simulink model "EGRVlv_VDPosGov"  (R2016b)
settings: configuration reference "CodeGenConfigSet" (kept outside this file)
values from neighbouring files (symbols this model uses):
  EGRVlv_ctClnUpFin_C = Calibration.Parameter    [init_EGRVlv_VDPosGov.m]
  EGRVlv_DKdNgv_C = Calibration.Parameter    [init_EGRVlv_VDPosGov.m]
  EGRVlv_DKdPsv_C = Calibration.Parameter    [init_EGRVlv_VDPosGov.m]
  EGRVlv_drActNgv_C = Calibration.Parameter    [init_EGRVlv_VDPosGov.m]
  EGRVlv_facCrntEffFlt_C = Calibration.Parameter    [init_EGRVlv_VDPosGov.m]
  EGRVlv_iEff_CUR = Calibration.Parameter    [init_EGRVlv_VDPosGov.m]
  EGRVlv_iEff_CURX = Calibration.Parameter    [init_EGRVlv_VDPosGov.m]
  EGRVlv_iEffOvrLd_C = Calibration.Parameter    [init_EGRVlv_VDPosGov.m]
  EGRVlv_IKiLMSSlp_C = Calibration.Parameter    [init_EGRVlv_VDPosGov.m]
  EGRVlv_IKiNgv_C = Calibration.Parameter    [init_EGRVlv_VDPosGov.m]
  EGRVlv_IKiPsv_C = Calibration.Parameter    [init_EGRVlv_VDPosGov.m]
  EGRVlv_KdParDT1_C = Calibration.Parameter    [init_EGRVlv_VDPosGov.m]
  EGRVlv_PKpNgv_C = Calibration.Parameter    [init_EGRVlv_VDPosGov.m]
  EGRVlv_PKpPsv_C = Calibration.Parameter    [init_EGRVlv_VDPosGov.m]
  EGRVlv_rActNgv_C = Calibration.Parameter    [init_EGRVlv_VDPosGov.m]
  EGRVlv_rDesClnUpCls_C = Calibration.Parameter    [init_EGRVlv_VDPosGov.m]
  EGRVlv_rDesClnUpOpen_C = Calibration.Parameter    [init_EGRVlv_VDPosGov.m]
  EGRVlv_rDesEGR_CUR = Calibration.Parameter    [init_EGRVlv_VDPosGov.m]
  EGRVlv_rDesEGR_CURX = Calibration.Parameter    [init_EGRVlv_VDPosGov.m]
  EGRVlv_rDesLMSMin_C = Calibration.Parameter    [init_EGRVlv_VDPosGov.m]
  EGRVlv_rDesOffHold_C = Calibration.Parameter    [init_EGRVlv_VDPosGov.m]
  EGRVlv_rEGRDflVal_C = Calibration.Parameter    [init_EGRVlv_VDPosGov.m]
  EGRVlv_rEGRSwtOff_C = Calibration.Parameter    [init_EGRVlv_VDPosGov.m]
  EGRVlv_rGovDvtThres_C = Calibration.Parameter    [init_EGRVlv_VDPosGov.m]
  EGRVlv_rGovMax_C = Calibration.Parameter    [init_EGRVlv_VDPosGov.m]
  EGRVlv_rGovMax_CUR = Calibration.Parameter    [init_EGRVlv_VDPosGov.m]
  EGRVlv_rGovMax_CURX = Calibration.Parameter    [init_EGRVlv_VDPosGov.m]
  EGRVlv_rGovMin_C = Calibration.Parameter    [init_EGRVlv_VDPosGov.m]
  EGRVlv_rGovMin_CUR = Calibration.Parameter    [init_EGRVlv_VDPosGov.m]
  EGRVlv_rGovMin_CURX = Calibration.Parameter    [init_EGRVlv_VDPosGov.m]
  EGRVlv_rIniStp_C = Calibration.Parameter    [init_EGRVlv_VDPosGov.m]
  EGRVlv_rOutDMax_C = Calibration.Parameter    [init_EGRVlv_VDPosGov.m]
  EGRVlv_rOutIMax_C = Calibration.Parameter    [init_EGRVlv_VDPosGov.m]
  EGRVlv_rPIDWinNgv_C = Calibration.Parameter    [init_EGRVlv_VDPosGov.m]
  EGRVlv_rPIDWinPsv_C = Calibration.Parameter    [init_EGRVlv_VDPosGov.m]
  EGRVlv_rSwtOffRmp_C = Calibration.Parameter    [init_EGRVlv_VDPosGov.m]
  EGRVlv_SlwClsDKd_C = Calibration.Parameter    [init_EGRVlv_VDPosGov.m]
  EGRVlv_SlwClsIKi_C = Calibration.Parameter    [init_EGRVlv_VDPosGov.m]
  EGRVlv_SlwClsPKp_C = Calibration.Parameter    [init_EGRVlv_VDPosGov.m]
  EGRVlv_SmlSigNgvDKd_C = Calibration.Parameter    [init_EGRVlv_VDPosGov.m]
  EGRVlv_SmlSigNgvIKi_C = Calibration.Parameter    [init_EGRVlv_VDPosGov.m]
  EGRVlv_SmlSigNgvPKp_C = Calibration.Parameter    [init_EGRVlv_VDPosGov.m]
  EGRVlv_SmlSigPsvDKd_C = Calibration.Parameter    [init_EGRVlv_VDPosGov.m]
  EGRVlv_SmlSigPsvIKi_C = Calibration.Parameter    [init_EGRVlv_VDPosGov.m]
  EGRVlv_SmlSigPsvPKp_C = Calibration.Parameter    [init_EGRVlv_VDPosGov.m]
  EGRVLV_STCLNUP_CLOSE = fi(3,State_uint8)    [init_EGRVlv_VDPosGov.m]
  EGRVLV_STCLNUP_FINISH = fi(4,State_uint8)    [init_EGRVlv_VDPosGov.m]
  EGRVLV_STCLNUP_INIT = fi(1,State_uint8)    [init_EGRVlv_VDPosGov.m]
  EGRVLV_STCLNUP_OPEN = fi(2,State_uint8)    [init_EGRVlv_VDPosGov.m]
  EGRVlv_stClnUpInh_C = Calibration.Parameter    [init_EGRVlv_VDPosGov.m]
  EGRVlv_swtDesValNrmInv_C = Calibration.Parameter    [init_EGRVlv_VDPosGov.m]
  EGRVlv_swtEGRTyp_C = Calibration.Parameter    [init_EGRVlv_VDPosGov.m]
  EGRVlv_swtGovByp_C = Calibration.Parameter    [init_EGRVlv_VDPosGov.m]
  EGRVlv_swtSelDT1In_C = Calibration.Parameter    [init_EGRVlv_VDPosGov.m]
  EGRVlv_tiClnUp_C = Calibration.Parameter    [init_EGRVlv_VDPosGov.m]
  EGRVlv_tiGovDT1_C = Calibration.Parameter    [init_EGRVlv_VDPosGov.m]
  EGRVlv_tiLimDlyOvrLd_C = Calibration.Parameter    [init_EGRVlv_VDPosGov.m]
  EGRVlv_tiOutIMax_C = Calibration.Parameter    [init_EGRVlv_VDPosGov.m]
  EGRVlv_tiParDT1_C = Calibration.Parameter    [init_EGRVlv_VDPosGov.m]
  MINUS_1_PRC = fi(-1,Prc_100_rate)    [init_EGRVlv_VDPosGov.m]
  RLS = fi(0,State_uint8)    [init_EGRVlv_VDPosGov.m]
  VALEO = fi(0,State_uint8)    [init_EGRVlv_VDPosGov.m]
  ZERO_PRC = fi(0,Prc_100_rate)    [init_EGRVlv_VDPosGov.m]
undefined symbols (not defined in the file or in its folder): CEngDsT_tTransf_CURX, EGRVlv_VDPosGov_DT, SubSysExeState_conv
libraries: CXLib x32, simulink x12
(part 2 of 2)

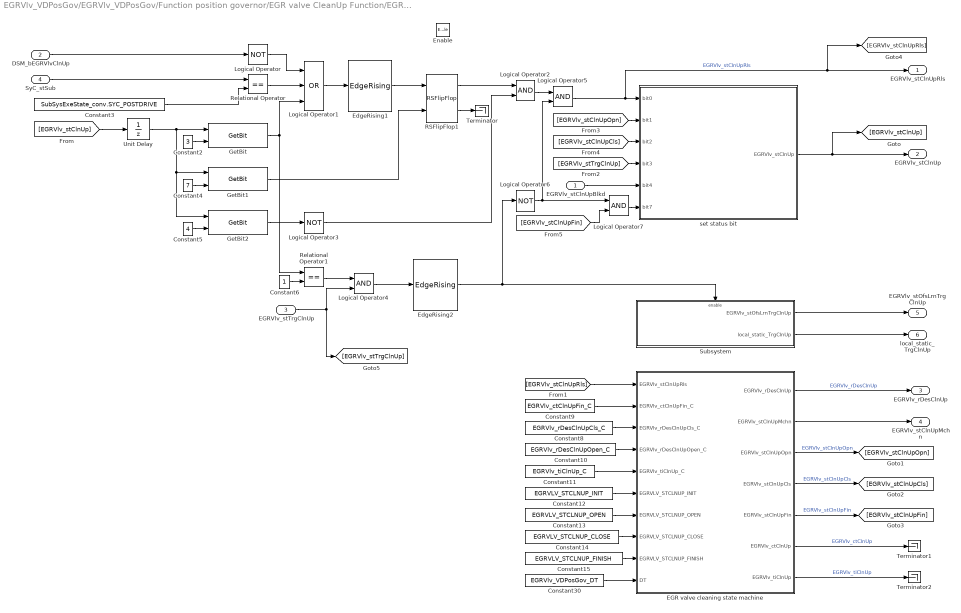
== system EGRVlv_VDPosGov/EGRVlv_VDPosGov/Function position governor/EGR valve CleanUp Function/EGR valve CleanUp release conditions ==
  EGRVlv_stClnUpBlkd : Inport
  DSM_bEGRVlvClnUp : Inport  Tag=%  Port=2
  EGRVlv_stTrgClnUp : Inport  Port=3
  SyC_stSub : Inport  Tag=%  Port=4
  Enable : EnablePort
  Constant10 : Constant  Value=EGRVlv_rDesClnUpOpen_C
  Constant11 : Constant  Value=EGRVlv_tiClnUp_C
  Constant12 : Constant  Value=EGRVLV_STCLNUP_INIT
  Constant13 : Constant  Value=EGRVLV_STCLNUP_OPEN
  Constant14 : Constant  Value=EGRVLV_STCLNUP_CLOSE
  Constant15 : Constant  Value=EGRVLV_STCLNUP_FINISH
  Constant2 : Constant  Value=3  OutDataTypeStr=uint8
  Constant3 : Constant  Value=SubSysExeState_conv.SYC_POSTDRIVE  OutDataTypeStr=Enum:SubSysExeState_conv
  Constant30 : Constant  Value=EGRVlv_VDPosGov_DT
  Constant4 : Constant  Value=7  OutDataTypeStr=uint8
  Constant5 : Constant  Value=4  OutDataTypeStr=uint8
  Constant6 : Constant  OutDataTypeStr=uint8
  Constant8 : Constant  Value=EGRVlv_rDesClnUpCls_C
  Constant9 : Constant  Value=EGRVlv_ctClnUpFin_C
  EGR valve cleaning state machine : Stateflow chart  TreatAsAtomicUnit=on
  EdgeRising1 : CXLib/EdgeRising
  EdgeRising2 : CXLib/EdgeRising
  GetBit : CXLib/GetBit  dataTypeString=uint8  dataLength=0
      settings: AttributesFormatString=Get bit from %<dataTypeString>
  GetBit1 : CXLib/GetBit  dataTypeString=uint8  dataLength=0
      settings: AttributesFormatString=Get bit from %<dataTypeString>
  GetBit2 : CXLib/GetBit  dataTypeString=uint8  dataLength=0
      settings: AttributesFormatString=Get bit from %<dataTypeString>
  Logical Operator : Logic  Operator=NOT  AllPortsSameDT=off  OutDataTypeStr=boolean
  Logical Operator1 : Logic  Operator=OR  Inputs=3  AllPortsSameDT=off  OutDataTypeStr=boolean
  Logical Operator{2,4..5,7} (4 alike) : Logic  AllPortsSameDT=off  OutDataTypeStr=boolean
  Logical Operator3 : Logic  Operator=NOT  AllPortsSameDT=off  OutDataTypeStr=boolean
  Logical Operator6 : Logic  Operator=NOT  AllPortsSameDT=off  OutDataTypeStr=boolean
  RSFlipFlop1 : CXLib/RSFlipFlop
  Relational Operator : RelationalOperator  Operator===  OutDataTypeStr=boolean  RndMeth=Simplest
  Relational Operator1 : RelationalOperator  Operator===  OutDataTypeStr=boolean  RndMeth=Simplest
  Subsystem : Subsystem
  Terminator : Terminator
  Terminator1 : Terminator
  Terminator2 : Terminator
  Unit Delay : UnitDelay  SampleTime=-1
      settings: AttributesFormatString=InitialValue=%<InitialCondition>
  set status bit : Subsystem
  EGRVlv_stClnUpRls : Outport  Tag=%
  EGRVlv_stClnUp : Outport  Tag=%  Port=2
  EGRVlv_rDesClnUp : Outport  Tag=%  Port=3
  EGRVlv_stClnUpMchn : Outport  Tag=%  Port=4
  EGRVlv_stOfsLrnTrgClnUp : Outport  Tag=%  Port=5
  local_static_TrgClnUp : Outport  Tag=%  Port=6
  wires:
  DSM_bEGRVlvClnUp/1 -> Logical Operator/1
  Logical Operator/1 -> Logical Operator1/1
  Logical Operator1/1 -> EdgeRising1/1
  EdgeRising1/1 -> RSFlipFlop1/1
  RSFlipFlop1/1 -> Logical Operator2/1
  Constant2/1 -> GetBit/2
  Constant3/1 -> Relational Operator/2
  SyC_stSub/1 -> Relational Operator/1
  GetBit/1 -> Logical Operator1/3, Relational Operator1/1
  Constant4/1 -> GetBit1/2
  GetBit1/1 -> RSFlipFlop1/2
  Constant5/1 -> GetBit2/2
  [EGRVlv_stClnUp] -> Unit Delay/1
  GetBit2/1 -> Logical Operator3/1
  Logical Operator3/1 -> Logical Operator2/2
  Relational Operator1/1 -> Logical Operator4/1
  Logical Operator4/1 -> EdgeRising2/1
  EdgeRising2/1 -> Subsystem/Enable, Logical Operator6/1
  EGRVlv_stTrgClnUp/1 -> [EGRVlv_stTrgClnUp], Logical Operator4/2
  Logical Operator2/1 -> Logical Operator5/1
  Constant6/1 -> Relational Operator1/2
  Logical Operator6/1 -> Logical Operator5/2, Logical Operator7/1
  Logical Operator5/1 -> [EGRVlv_stClnUpRls], EGRVlv_stClnUpRls/1, set status bit/1(bit0)  "EGRVlv_stClnUpRls"
  Constant9/1 -> EGR valve cleaning state machine/2(EGRVlv_ctClnUpFin_C)
  Constant8/1 -> EGR valve cleaning state machine/3(EGRVlv_rDesClnUpCls_C)
  Constant10/1 -> EGR valve cleaning state machine/4(EGRVlv_rDesClnUpOpen_C)
  Constant11/1 -> EGR valve cleaning state machine/5(EGRVlv_tiClnUp_C)
  Constant30/1 -> EGR valve cleaning state machine/10(DT)
  set status bit/1(EGRVlv_stClnUp) -> [EGRVlv_stClnUp], EGRVlv_stClnUp/1
  Logical Operator7/1 -> set status bit/6(bit7)
  [EGRVlv_stClnUpFin] -> Logical Operator7/2
  Constant12/1 -> EGR valve cleaning state machine/6(EGRVLV_STCLNUP_INIT)
  Constant13/1 -> EGR valve cleaning state machine/7(EGRVLV_STCLNUP_OPEN)
  Constant15/1 -> EGR valve cleaning state machine/9(EGRVLV_STCLNUP_FINISH)
  Constant14/1 -> EGR valve cleaning state machine/8(EGRVLV_STCLNUP_CLOSE)
  Relational Operator/1 -> Logical Operator1/2
  Unit Delay/1 -> GetBit/1, GetBit2/1, GetBit1/1
  [EGRVlv_stClnUpRls] -> EGR valve cleaning state machine/1(EGRVlv_stClnUpRls)
  [EGRVlv_stClnUpOpn] -> set status bit/2(bit1)
  [EGRVlv_stClnUpCls] -> set status bit/3(bit2)
  [EGRVlv_stTrgClnUp] -> set status bit/4(bit3)
  EGRVlv_stClnUpBlkd/1 -> set status bit/5(bit4)
  EGR valve cleaning state machine/1(EGRVlv_rDesClnUp) -> EGRVlv_rDesClnUp/1  "EGRVlv_rDesClnUp"
  EGR valve cleaning state machine/2(EGRVlv_stClnUpMchn) -> EGRVlv_stClnUpMchn/1
  EGR valve cleaning state machine/3(EGRVlv_stClnUpOpn) -> [EGRVlv_stClnUpOpn]  "EGRVlv_stClnUpOpn"
  EGR valve cleaning state machine/4(EGRVlv_stClnUpCls) -> [EGRVlv_stClnUpCls]  "EGRVlv_stClnUpCls"
  EGR valve cleaning state machine/5(EGRVlv_stClnUpFin) -> [EGRVlv_stClnUpFin]  "EGRVlv_stClnUpFin"
  EGR valve cleaning state machine/6(EGRVlv_ctClnUp) -> Terminator1/1  "EGRVlv_ctClnUp"
  EGR valve cleaning state machine/7(EGRVlv_tiClnUp) -> Terminator2/1  "EGRVlv_tiClnUp"
  RSFlipFlop1/2 -> Terminator/1
  Subsystem/1(EGRVlv_stOfsLrnTrgClnUp) -> EGRVlv_stOfsLrnTrgClnUp/1
  Subsystem/2(local_static_TrgClnUp) -> local_static_TrgClnUp/1

== system EGRVlv_VDPosGov/EGRVlv_VDPosGov/Function position governor/EGR valve CleanUp Function/Subsystem1 ==
  Enable : EnablePort
  Constant1 : Constant  Value=0  OutDataTypeStr=boolean
  Constant7 : Constant  OutDataTypeStr=boolean
  EGRVlv_stOfsLrnTrgClnUp : Outport  Tag=%
  local_static_TrgClnUp : Outport  Tag=%  Port=2
  wires:
  Constant1/1 -> local_static_TrgClnUp/1
  Constant7/1 -> EGRVlv_stOfsLrnTrgClnUp/1

== system EGRVlv_VDPosGov/EGRVlv_VDPosGov/Function position governor/I_comp/Calc ==
  note: %系数Q=Ki*T0/100
  note: [Dvt/s]
  note: [Dvt/ms]
  Dvt : Inport
  T0 : Inport  Port=2
  Ki : Inport  Port=3
  KiPos : Inport  Port=4
  KiNeg : Inport  Port=5
  WinPos : Inport  Port=6
  WinNeg : Inport  Port=7
  function : TriggerPort  TriggerType=function-call  VariantControl=Variant
  Constant1 : Constant  Value=100  OutDataTypeStr=uint32
  Data Store Read : DataStoreRead  DataStoreName=outputlast1
  Data Store Write : DataStoreWrite  DataStoreName=outputlast1
  Data Type Conversion11 : DataTypeConversion  SaturateOnIntegerOverflow=on
  Divide2 : Product  Inputs=*/  OutDataTypeStr=fixdt(1,32,2^-16,0)  RndMeth=Round  SaturateOnIntegerOverflow=on
  Product1 : Product  OutDataTypeStr=fixdt(1,32,2^-16,0)  RndMeth=Round  SaturateOnIntegerOverflow=on
  Product3 : Product  OutDataTypeStr=fixdt(1,32,2^-16,0)  RndMeth=Round  SaturateOnIntegerOverflow=on
  Relational Operator : RelationalOperator  Operator=>  OutDataTypeStr=boolean  RndMeth=Nearest  InputSameDT=on
  Relational Operator1 : RelationalOperator  Operator=<  OutDataTypeStr=boolean  RndMeth=Nearest  InputSameDT=on
  Sum : Sum  OutDataTypeStr=fixdt(1,32,2^-16,0)  RndMeth=Round  SaturateOnIntegerOverflow=on  InputSameDT=on
  Switch : Switch  Criteria=u2 ~= 0  SaturateOnIntegerOverflow=on  InputSameDT=on
  Switch1 : Switch  Criteria=u2 ~= 0  SaturateOnIntegerOverflow=on  InputSameDT=on
  Out : Outport
  wires:
  Product3/1 -> Sum/2
  Divide2/1 -> Product3/2
  Constant1/1 -> Divide2/2
  Product1/1 -> Divide2/1
  Data Type Conversion11/1 -> Out/1
  Sum/1 -> Data Type Conversion11/1, Data Store Write/1
  Dvt/1 -> Relational Operator1/1, Relational Operator/1, Product3/1
  Switch1/1 -> Product1/1
  T0/1 -> Product1/2
  WinNeg/1 -> Relational Operator1/2
  Ki/1 -> Switch/3
  Data Store Read/1 -> Sum/1
  Switch/1 -> Switch1/3
  WinPos/1 -> Relational Operator/2
  Relational Operator1/1 -> Switch/2
  KiNeg/1 -> Switch/1
  Relational Operator/1 -> Switch1/2
  KiPos/1 -> Switch1/1

== system EGRVlv_VDPosGov/EGRVlv_VDPosGov/Function position governor/I_comp/Init ==
  InitVal : Inport
  function : TriggerPort  TriggerType=function-call  VariantControl=Variant
  Constant2 : Constant  OutDataTypeStr=uint32
  Data Store Write : DataStoreWrite  DataStoreName=outputlast1
  Divide1 : Product  Inputs=**  OutDataTypeStr=Inherit: Inherit via back propagation  RndMeth=Round  SaturateOnIntegerOverflow=on
  wires:
  Constant2/1 -> Divide1/2
  Divide1/1 -> Data Store Write/1
  InitVal/1 -> Divide1/1

== system EGRVlv_VDPosGov/EGRVlv_VDPosGov/Function position governor/Switch Governor Output/Initialisation of EGRVlv_swtEGRTyp ==
  Constant5 : Constant  Value=EGRVlv_swtEGRTyp_C
  Constant6 : Constant  Value=15  OutDataTypeStr=Inherit: Inherit via back propagation
  Relational Operator : RelationalOperator  Operator=~=  OutDataTypeStr=boolean  RndMeth=Simplest  InputSameDT=on
  Switch1 : Switch  Criteria=u2 ~= 0
  Unit Delay1 : UnitDelay  SampleTime=-1
      settings: AttributesFormatString=InitialValue=%<InitialCondition>
  EGRVlv_swtEGRTyp : Outport  Tag=%
  wires:
  Switch1/1 -> EGRVlv_swtEGRTyp/1, Unit Delay1/1
  Constant6/1 -> Relational Operator/2
  Unit Delay1/1 -> Switch1/3
  Relational Operator/1 -> Switch1/2
  Constant5/1 -> Switch1/1, Relational Operator/1

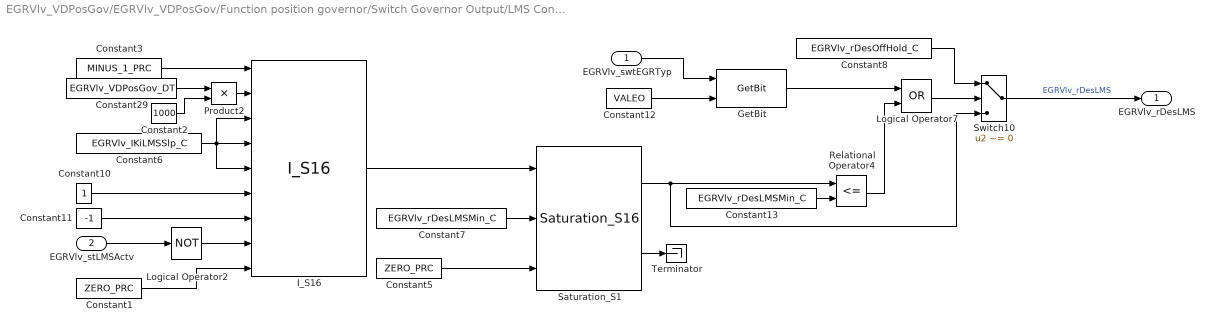
== system EGRVlv_VDPosGov/EGRVlv_VDPosGov/Function position governor/Switch Governor Output/LMS Control ==
  EGRVlv_swtEGRTyp : Inport  Tag=%
  EGRVlv_stLMSActv : Inport  Tag=%  Port=2
  Constant1 : Constant  Value=ZERO_PRC
  Constant10 : Constant  OutDataTypeStr=Prc_100_rate
  Constant11 : Constant  Value=-1  OutDataTypeStr=Prc_100_rate
  Constant12 : Constant  Value=VALEO
  Constant13 : Constant  Value=EGRVlv_rDesLMSMin_C
  Constant2 : Constant  Value=1000  OutDataTypeStr=uint16
  Constant29 : Constant  Value=EGRVlv_VDPosGov_DT
  Constant3 : Constant  Value=MINUS_1_PRC
  Constant5 : Constant  Value=ZERO_PRC
  Constant6 : Constant  Value=EGRVlv_IKiLMSSlp_C
  Constant7 : Constant  Value=EGRVlv_rDesLMSMin_C
  Constant8 : Constant  Value=EGRVlv_rDesOffHold_C
  GetBit : CXLib/GetBit  dataTypeString=uint8  dataLength=0
      settings: AttributesFormatString=Get bit from %<dataTypeString>
  I_S16 : CXLib/I_S16
  Logical Operator2 : Logic  Operator=NOT  AllPortsSameDT=off  OutDataTypeStr=boolean
  Logical Operator7 : Logic  Operator=OR  AllPortsSameDT=off  OutDataTypeStr=boolean
  Product2 : Product  OutDataTypeStr=Inherit: Inherit via back propagation  SaturateOnIntegerOverflow=on
  Relational Operator4 : RelationalOperator  Operator=<=  OutDataTypeStr=boolean  RndMeth=Simplest
  Saturation_S1 : CXLib/Saturation_S16
  Switch10 : Switch  Criteria=u2 ~= 0
  Terminator : Terminator
  EGRVlv_rDesLMS : Outport  Tag=%
  wires:
  Constant8/1 -> Switch10/1
  Constant3/1 -> I_S16/1
  Relational Operator4/1 -> Logical Operator7/2
  Constant5/1 -> Saturation_S1/3
  Logical Operator7/1 -> Switch10/2
  Constant7/1 -> Saturation_S1/2
  GetBit/1 -> Logical Operator7/1
  Constant13/1 -> Relational Operator4/2
  Switch10/1 -> EGRVlv_rDesLMS/1  "EGRVlv_rDesLMS"
  Constant1/1 -> I_S16/9
  Constant10/1 -> I_S16/6
  Constant6/1 -> I_S16/3, I_S16/5, I_S16/4
  Constant11/1 -> I_S16/7
  I_S16/1 -> Saturation_S1/1
  Saturation_S1/1 -> Relational Operator4/1, Switch10/3
  Constant12/1 -> GetBit/2
  EGRVlv_swtEGRTyp/1 -> GetBit/1
  EGRVlv_stLMSActv/1 -> Logical Operator2/1
  Saturation_S1/2 -> Terminator/1
  Logical Operator2/1 -> I_S16/8
  Constant29/1 -> Product2/1
  Product2/1 -> I_S16/2
  Constant2/1 -> Product2/2

== system EGRVlv_VDPosGov/EGRVlv_VDPosGov/Function position governor/EGR valve CleanUp Function/EGR valve CleanUp release conditions/Subsystem ==
  Enable : EnablePort
  Constant1 : Constant  OutDataTypeStr=boolean
  Constant7 : Constant  Value=0  OutDataTypeStr=boolean
  EGRVlv_stOfsLrnTrgClnUp : Outport  Tag=%
  local_static_TrgClnUp : Outport  Tag=%  Port=2
  wires:
  Constant1/1 -> local_static_TrgClnUp/1
  Constant7/1 -> EGRVlv_stOfsLrnTrgClnUp/1

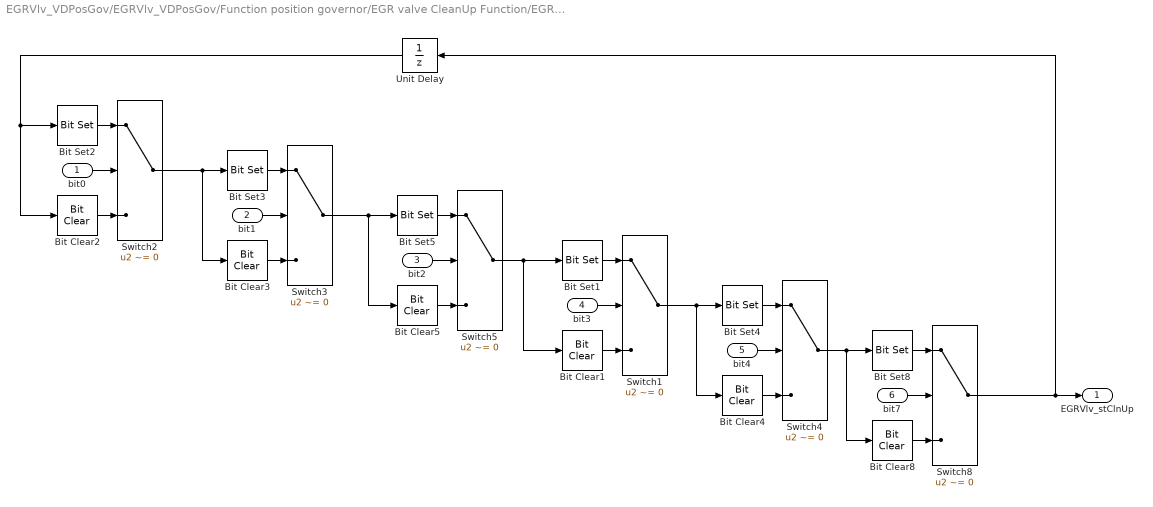
== system EGRVlv_VDPosGov/EGRVlv_VDPosGov/Function position governor/EGR valve CleanUp Function/EGR valve CleanUp release conditions/set status bit ==
  bit0 : Inport
  bit1 : Inport  Port=2
  bit2 : Inport  Port=3
  bit3 : Inport  Port=4
  bit4 : Inport  Port=5
  bit7 : Inport  Port=6
  Bit Clear1 : simulink/Logic and Bit Operations/Bit Clear  iBit=3
  Bit Clear2 : simulink/Logic and Bit Operations/Bit Clear  iBit=0
  Bit Clear3 : simulink/Logic and Bit Operations/Bit Clear  iBit=1
  Bit Clear4 : simulink/Logic and Bit Operations/Bit Clear  iBit=4
  Bit Clear5 : simulink/Logic and Bit Operations/Bit Clear  iBit=2
  Bit Clear8 : simulink/Logic and Bit Operations/Bit Clear  iBit=7
  Bit Set1 : simulink/Logic and Bit Operations/Bit Set  iBit=3
  Bit Set2 : simulink/Logic and Bit Operations/Bit Set  iBit=0
  Bit Set3 : simulink/Logic and Bit Operations/Bit Set  iBit=1
  Bit Set4 : simulink/Logic and Bit Operations/Bit Set  iBit=4
  Bit Set5 : simulink/Logic and Bit Operations/Bit Set  iBit=2
  Bit Set8 : simulink/Logic and Bit Operations/Bit Set  iBit=7
  Switch{1..5,8} (6 alike) : Switch  Criteria=u2 ~= 0  OutDataTypeStr=Inherit: Inherit via back propagation  SaturateOnIntegerOverflow=on  InputSameDT=on
  Unit Delay : UnitDelay  SampleTime=-1
      settings: AttributesFormatString=InitialValue=%<InitialCondition>
  EGRVlv_stClnUp : Outport
  wires:
  bit7/1 -> Switch8/2
  Bit Clear8/1 -> Switch8/3
  Bit Set8/1 -> Switch8/1
  bit2/1 -> Switch5/2
  Bit Clear5/1 -> Switch5/3
  Bit Set5/1 -> Switch5/1
  Switch8/1 -> Unit Delay/1, EGRVlv_stClnUp/1
  bit1/1 -> Switch3/2
  Switch2/1 -> Bit Set3/1, Bit Clear3/1
  Bit Clear3/1 -> Switch3/3
  Bit Set3/1 -> Switch3/1
  bit0/1 -> Switch2/2
  Bit Clear2/1 -> Switch2/3
  Bit Set2/1 -> Switch2/1
  Switch3/1 -> Bit Clear5/1, Bit Set5/1
  Unit Delay/1 -> Bit Clear2/1, Bit Set2/1
  bit3/1 -> Switch1/2
  Bit Clear1/1 -> Switch1/3
  Bit Set1/1 -> Switch1/1
  Switch5/1 -> Bit Clear1/1, Bit Set1/1
  bit4/1 -> Switch4/2
  Bit Clear4/1 -> Switch4/3
  Bit Set4/1 -> Switch4/1
  Switch1/1 -> Bit Clear4/1, Bit Set4/1
  Switch4/1 -> Bit Clear8/1, Bit Set8/1

== stateflow chart EGRVlv_VDPosGov/Function position governor/EGR valve CleanUp Function/EGR valve CleanUp release conditions/EGR valve cleaning state machine ==
  state EGRVLV_STCLNUP_INIT
    entry: EGRVlv_ctClnUp = 0;
    EGRVlv_tiClnUp = 0;
    EGRVlv_stClnUpMchn = EGRVLV_STCLNUP_INIT;
  state EGRVLV_STCLNUP
    state EGRVLV_STCLNUP_OPEN
      entry:
      EGRVlv_stClnUpOpn = 1;
      EGRVlv_rDesClnUp = EGRVlv_rDesClnUpOpen_C;
      EGRVlv_stClnUpMchn = EGRVLV_STCLNUP_OPEN;
      during:
      EGRVlv_tiClnUp = EGRVlv_tiClnUp + DT;
      exit:
      EGRVlv_tiClnUp = 0;
      EGRVlv_stClnUpOpn = 0;
    state EGRVLV_STCLNUP_CLOSE
      entry:
      EGRVlv_stClnUpCls = 1;
      EGRVlv_rDesClnUp = EGRVlv_rDesClnUpCls_C;
      EGRVlv_ctClnUp = EGRVlv_ctClnUp + 1;
      EGRVlv_stClnUpMchn = EGRVLV_STCLNUP_CLOSE;
      during:
      EGRVlv_tiClnUp = EGRVlv_tiClnUp + DT;
      exit: EGRVlv_tiClnUp = 0;
      EGRVlv_stClnUpCls = 0;
    state EGRVLV_STCLNUP_FINISH
      entry:  EGRVlv_stClnUpFin = 1;
      EGRVlv_rDesClnUp = 0;
      EGRVlv_ctClnUp = 0;
      EGRVlv_stClnUpMchn = EGRVLV_STCLNUP_FINISH;
    (default) -> EGRVLV_STCLNUP_OPEN
    EGRVLV_STCLNUP_CLOSE -> EGRVLV_STCLNUP_OPEN [order 1] : [(EGRVlv_tiClnUp >= EGRVlv_tiClnUp_C)&&...
        | (EGRVlv_ctClnUp < EGRVlv_ctClnUpFin_C)]
    EGRVLV_STCLNUP_OPEN -> EGRVLV_STCLNUP_CLOSE : [EGRVlv_tiClnUp >= EGRVlv_tiClnUp_C]
    EGRVLV_STCLNUP_CLOSE -> EGRVLV_STCLNUP_FINISH [order 2] : [(EGRVlv_tiClnUp >= EGRVlv_tiClnUp_C)&&...
        | (EGRVlv_ctClnUp >= EGRVlv_ctClnUpFin_C)]
  (default) -> EGRVLV_STCLNUP_INIT
  EGRVLV_STCLNUP -> EGRVLV_STCLNUP_INIT : [EGRVlv_stClnUpRls==0]
  EGRVLV_STCLNUP_INIT -> EGRVLV_STCLNUP : [EGRVlv_stClnUpRls==1]
  data: EGRVlv_stClnUpRls input; EGRVlv_ctClnUpFin_C input; EGRVlv_rDesClnUpCls_C input; EGRVlv_rDesClnUpOpen_C input; EGRVlv_tiClnUp_C input; EGRVLV_STCLNUP_INIT input; EGRVLV_STCLNUP_OPEN input; EGRVlv_rDesClnUp output; EGRVlv_stClnUpMchn output; EGRVlv_stClnUpOpn output; EGRVLV_STCLNUP_CLOSE input; EGRVLV_STCLNUP_FINISH input; DT input; EGRVlv_stClnUpCls output; EGRVlv_stClnUpFin output; EGRVlv_ctClnUp output Counter_num; EGRVlv_tiClnUp output Debounce_ms
